simulink model "MSE452_Lab2_CHB_samplemodel"  (R2023a)
settings: Solver=ode23t  StartTime=0.0  StopTime=0.1  MaxStep=1e-5  RelTol=1e-3  EnableMultiTasking=on
InitFcn:
  | ma=0.99
  | f1=60
  | T1=1/f1
  | fs_ps=720
  | Ts_ps=1/fs_ps
  | fs_ls=4320
  | Ts_ls=1/fs_ls
values from neighbouring files (symbols this model uses):
  E = ratedOutputVoltage/3    (= 766.666666667)    [main.m]
  L = X / (2 * pi * ratedOutputFrequency)    [main.m]
  R = real(Z)    [main.m]
libraries: spsDCVoltageSourceLib x9, spsUniversalBridgeLib x9, spsTriangleGeneratorLib x9, spsVoltageMeasurementLib x5, spsSeriesRLCBranchLib x3, simulink x1, sps_lib x1
settings Model: Creator=jw  LastModifiedBy=auamai
settings SolverCC: AlgebraicLoopSolver=TrustRegion
settings DataIOCC: LimitDataPoints=on  SaveFormat=Array  SignalLoggingSaveFormat=ModelDataLogs  ReturnWorkspaceOutputs=off
settings OptimizationCC: InitFltsAndDblsToZero=on  LifeSpan=inf
settings DebuggingCC: SaveWithParameterizedLinksMsg=none  UnderspecifiedInitializationDetection=Classic  MergeDetectMultiDrivingBlocksExec=none  SignalResolutionControl=TryResolveAllWithWarning  SolverPrmCheckMsg=warning  MultiTaskDSMMsg=warning  MultiTaskCondExecSysMsg=none  FcnCallInpInsideContextMsg=warning  UnconnectedInputMsg=warning  UnconnectedOutputMsg=warning  UnconnectedLineMsg=warning  SFUnexpectedBacktrackingDiag=warning  SFNoUnconditionalDefaultTransitionDiag=warning  SFExecutionAtInitializationDiag=none  ArithmeticOperatorsInVariantConditions=warning
settings HardwareCC: ProdBitPerPointer=32  ProdBitPerSizeT=32  ProdBitPerPtrDiffT=32  ProdLargestAtomicFloat=None  ProdIntDivRoundTo=Undefined  ProdEndianess=Unspecified  ProdWordSize=32  ProdHWDeviceType=32-bit Generic
settings ModelReferenceCC: EnableRefExpFcnMdlSchedulingChecks=on  PropagateSignalLabelsOutOfModel=off
settings SFSimCC: CustomCodeUndefinedFunction=UseInterfaceOnly
settings CodeAppCC: StateflowObjectComments=on
settings GRTTargetCC: TargetFcnLib=ansi_tfl_tmw.mat  TargetLangStandard=C89/C90 (ANSI)  CombineOutputUpdateFcns=off  GRTInterface=on
settings ConfigComp: CovMetricSettings=dw  CovSaveCumulativeToWorkspaceVar=on  CovSaveSingleToWorkspaceVar=on

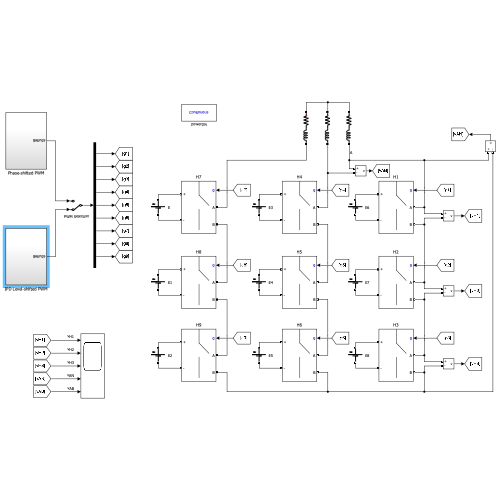
[thumbnail: Simulink's stored preview of the top-level diagram]
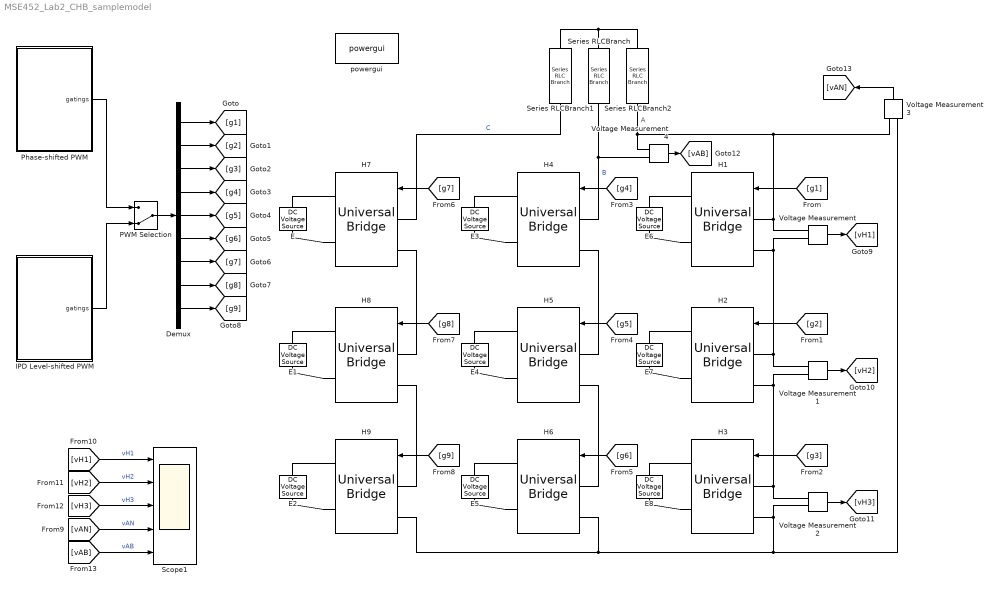
== system MSE452_Lab2_CHB_samplemodel ==
  note: A
  Demux : Demux  Outputs=9
  E{,1..8} (9 alike) : spsDCVoltageSourceLib/DC Voltage Source  Amplitude=E  Measurements=None
  H{1..9} (9 alike) : spsUniversalBridgeLib/Universal Bridge  Arms=2  SnubberResistance=1e5  SnubberCapacitance=inf  Device=Ideal Switches  Ron=1e-3  Lon=0  ForwardVoltages="[  0  0  ]"  ForwardVoltage=0  GTOparameters=[ 10e-6 , 20e-6 ]  IGBTparameters=[ 1e-6 , 2e-6 ]  Measurements=None  Measurements_2=None  converterType=Rectifier
  IPD Level-shifted PWM : Subsystem
  PWM Selection : ManualSwitch  CurrentSetting=0
  Phase-shifted PWM : Subsystem
  Scope1 : Scope  NumInputPorts=5
  Series RLCBranch : spsSeriesRLCBranchLib/Series RLC Branch  LConnTagsString=__new0  RConnTagsString=__new0  BranchType=RL  Resistance=R  Inductance=L  SetiL0=off  InitialCurrent=0  Capacitance=1e-6  Setx0=off  InitialVoltage=0  Measurements=None
  Series RLCBranch1 : spsSeriesRLCBranchLib/Series RLC Branch  LConnTagsString=__new0  RConnTagsString=__new0  BranchType=RL  Resistance=R  Inductance=L  SetiL0=off  InitialCurrent=0  Capacitance=1e-6  Setx0=off  InitialVoltage=0  Measurements=None
  Series RLCBranch2 : spsSeriesRLCBranchLib/Series RLC Branch  LConnTagsString=__new0  RConnTagsString=__new0  BranchType=RL  Resistance=R  Inductance=L  SetiL0=off  InitialCurrent=0  Capacitance=1e-6  Setx0=off  InitialVoltage=0  Measurements=None
  Voltage Measurement{,1..4} (5 alike) : spsVoltageMeasurementLib/Voltage Measurement  PhasorSimulation=off  OutputType=Complex  PSBequivalent=0
  powergui : sps_lib/powergui  Priority=1  SimulationMode=Continuous  SampleTime=50e-6  frequency=60  Iterations=50  frequencyindice=0  Pbase=100e6  ErrMax=1e-4  UnitsV=kV  UnitsW=MW  buscounter=0  FunctionMessages=off  echomessages=off  EnableUseOfTLC=off  CurrentSourceSwitches=off  DisableSnubberDevices=off  DisableRonSwitches=off  DisableVfSwitches=off  DisplayEquations=off  AutomaticDiscreteSolvers=off  SolverType=Tustin/Backward Euler (TBE)  Interpol=off  ExternalGateDelay=off  methode=off  Ts=100  x0status=blocks  SPID=on  SwTol=0  HookPort=off  NonlinearTolerance=1e-4  nMaxIteration=100  ContinueOnMaxIteration=off  RestoreLinks=warning  ResistiveCurrentMeasurement=off  Frange=[0:2:500]  Ylog=off  Xlog=on  ShowGrid=off  save=off  variable=ZData  structure=0  ZoomFFT=off  StartTime=0.0  cycles=1  DisplayStyle=1  fundamental=60  FreqAxis=off  MaxFrequency=1000  frequencyindicesteady=1  RmsSteady=1  display=off
  wires:
  [g1] -> H1/1
  [g2] -> H2/1
  [g3] -> H3/1
  [g4] -> H4/1
  [g5] -> H5/1
  [g6] -> H6/1
  [g7] -> H7/1
  [g8] -> H8/1
  [g9] -> H9/1
  Demux/1 -> [g1]
  Demux/2 -> [g2]
  Demux/3 -> [g3]
  Demux/4 -> [g4]
  Demux/5 -> [g5]
  Demux/6 -> [g6]
  Demux/7 -> [g7]
  Demux/8 -> [g8]
  Demux/9 -> [g9]
  Phase-shifted PWM/1(gatings) -> PWM Selection/1
  PWM Selection/1 -> Demux/1
  Voltage Measurement/1 -> [vH1]
  Voltage Measurement1/1 -> [vH2]
  Voltage Measurement2/1 -> [vH3]
  Voltage Measurement4/1 -> [vAB]
  Voltage Measurement3/1 -> [vAN]
  [vAN] -> Scope1/4  "vAN"
  [vH1] -> Scope1/1  "vH1"
  [vH2] -> Scope1/2  "vH2"
  [vH3] -> Scope1/3  "vH3"
  [vAB] -> Scope1/5  "vAB"
  IPD Level-shifted PWM/1(gatings) -> PWM Selection/2
  connections:
  H7/RConn2 -- E/LConn1
  E/RConn1 -- H7/RConn1
  E1/RConn1 -- H8/RConn1
  H8/RConn2 -- E1/LConn1
  E2/RConn1 -- H9/RConn1
  H9/RConn2 -- E2/LConn1
  H4/RConn2 -- E3/LConn1
  E5/RConn1 -- H6/RConn1
  E3/RConn1 -- H4/RConn1
  H6/RConn2 -- E5/LConn1
  E4/RConn1 -- H5/RConn1
  H5/RConn2 -- E4/LConn1
  H1/RConn2 -- E6/LConn1
  E8/RConn1 -- H3/RConn1
  E6/RConn1 -- H1/RConn1
  H3/RConn2 -- E8/LConn1
  E7/RConn1 -- H2/RConn1
  H2/RConn2 -- E7/LConn1
  H9/LConn2 -- H6/LConn2 -- H3/LConn2 -- Voltage Measurement2/LConn2 -- Voltage Measurement3/LConn2
  H9/LConn1 -- H8/LConn2
  H8/LConn1 -- H7/LConn2
  H4/LConn2 -- H5/LConn1
  H5/LConn2 -- H6/LConn1
  H1/LConn2 -- Voltage Measurement/LConn2 -- H2/LConn1 -- Voltage Measurement1/LConn1
  H2/LConn2 -- Voltage Measurement1/LConn2 -- H3/LConn1 -- Voltage Measurement2/LConn1
  H7/LConn1 -- Series RLCBranch1/RConn1  "C"
  Series RLCBranch/RConn1 -- H4/LConn1 -- Voltage Measurement4/LConn2  "B"
  H1/LConn1 -- Voltage Measurement/LConn1 -- Voltage Measurement3/LConn1 -- Series RLCBranch2/RConn1 -- Voltage Measurement4/LConn1
  Series RLCBranch1/LConn1 -- Series RLCBranch2/LConn1 -- Series RLCBranch/LConn1

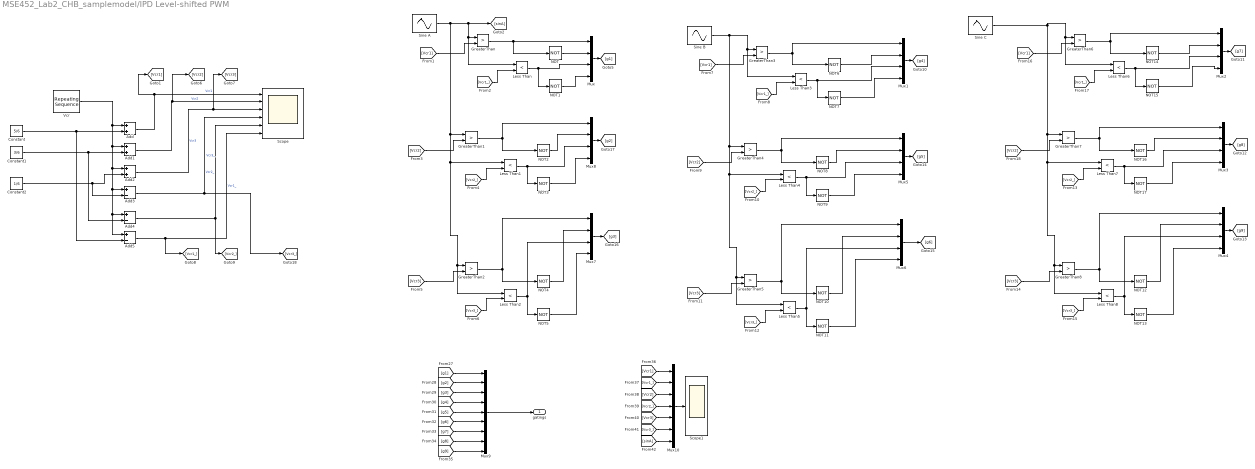
== system MSE452_Lab2_CHB_samplemodel/IPD Level-shifted PWM ==
  Add : Sum
  Add1 : Sum
  Add2 : Sum
  Add3 : Sum  Inputs=+-
  Add4 : Sum  Inputs=+-
  Add5 : Sum  Inputs=+-
  Constant : Constant  Value=5/6
  Constant1 : Constant  Value=3/6
  Constant2 : Constant  Value=1/6
  GreaterThan{,1..8} (9 alike) : RelationalOperator  Operator=>  OutDataTypeStr=boolean  RndMeth=Simplest  InputSameDT=off
  Less Than{,1..8} (9 alike) : RelationalOperator  Operator=<  OutDataTypeStr=boolean  RndMeth=Simplest  InputSameDT=off
  Mux{,1..8} (9 alike) : Mux
  Mux10 : Mux  Inputs=7
  Mux9 : Mux  Inputs=9
  NOT{,1..17} (18 alike) : Logic  Operator=NOT  IconShape=distinctive  AllPortsSameDT=off  OutDataTypeStr=boolean
  Scope : Scope  NumInputPorts=6
  Scope1 : Scope
  Sine A : Sin  Amplitude=0.25  Frequency=2*pi*f1  SampleTime=0
  Sine B : Sin  Amplitude=0.25  Frequency=2*pi*f1  Phase=-2/3*pi  SampleTime=0
  Sine C : Sin  Amplitude=0.25  Frequency=2*pi*f1  Phase=2/3*pi  SampleTime=0
  Vcr : simulink/Sources/Repeating Sequence  rep_seq_t=[0 1/4*Ts_ls 3/4*Ts_ls Ts_ls]  rep_seq_y=[0 1/6 -1/6 0]
  gatings : Outport  VectorParamsAs1DForOutWhenUnconnected=off
  wires:
  Mux9/1 -> gatings/1
  Mux/1 -> [g1]
  Mux1/1 -> [g4]
  Mux2/1 -> [g7]
  Mux3/1 -> [g8]
  Mux4/1 -> [g9]
  Mux5/1 -> [g5]
  Mux6/1 -> [g6]
  Mux7/1 -> [g3]
  Mux8/1 -> [g2]
  [g1] -> Mux9/1
  [g2] -> Mux9/2
  [g3] -> Mux9/3
  [g4] -> Mux9/4
  [g5] -> Mux9/5
  [g6] -> Mux9/6
  [g7] -> Mux9/7
  [g8] -> Mux9/8
  [g9] -> Mux9/9
  [Vcr1] -> Mux10/1
  [Vcr1_] -> Mux10/2
  [Vcr2] -> Mux10/3
  [Vcr2_] -> Mux10/4
  [Vcr3] -> Mux10/5
  [Vcr3_] -> Mux10/6
  Mux10/1 -> Scope1/1
  [sinA] -> Mux10/7
  Vcr/1 -> Add5/1, Add4/1, Add3/1, Add2/1, Add1/1, Add/1
  Constant/1 -> Add5/2, Add/2
  Add/1 -> [Vcr1], Scope/1  "Vcr1"
  Constant1/1 -> Add4/2, Add1/2
  Add1/1 -> [Vcr2], Scope/2  "Vcr2"
  Constant2/1 -> Add3/2, Add2/2
  Add2/1 -> [Vcr3], Scope/3  "Vcr3"
  Add5/1 -> [Vcr1_], Scope/6  "Vcr1_"
  Add3/1 -> [Vcr3_], Scope/4  "Vcr3_"
  Add4/1 -> [Vcr2_], Scope/5  "Vcr2_"
  [Vcr1] -> GreaterThan/2
  GreaterThan/1 -> NOT/1, Mux/1
  NOT/1 -> Mux/2
  [Vcr1_] -> Less Than/2
  Less Than/1 -> NOT1/1, Mux/3
  NOT1/1 -> Mux/4
  NOT2/1 -> Mux8/2
  [Vcr2_] -> Less Than1/2
  NOT3/1 -> Mux8/4
  Less Than1/1 -> Mux8/3, NOT3/1
  GreaterThan1/1 -> Mux8/1, NOT2/1
  [Vcr2] -> GreaterThan1/2
  GreaterThan2/1 -> Mux7/1, NOT4/1
  Less Than2/1 -> Mux7/3, NOT5/1
  [Vcr3_] -> Less Than2/2
  NOT5/1 -> Mux7/4
  [Vcr3] -> GreaterThan2/2
  Sine A/1 -> Less Than/1, GreaterThan/1, [sinA], Less Than1/1, Less Than2/1, GreaterThan2/1, GreaterThan1/1
  NOT4/1 -> Mux7/2
  NOT6/1 -> Mux1/2
  NOT11/1 -> Mux6/4
  Less Than5/1 -> Mux6/3, NOT11/1
  GreaterThan3/1 -> Mux1/1, NOT6/1
  Less Than4/1 -> Mux5/3, NOT9/1
  GreaterThan5/1 -> Mux6/1, NOT10/1
  [Vcr3] -> GreaterThan5/2
  [Vcr1_] -> Less Than3/2
  [Vcr2_] -> Less Than4/2
  [Vcr3_] -> Less Than5/2
  NOT10/1 -> Mux6/2
  [Vcr2] -> GreaterThan4/2
  Sine B/1 -> Less Than3/1, GreaterThan3/1, Less Than4/1, Less Than5/1, GreaterThan5/1, GreaterThan4/1
  GreaterThan4/1 -> Mux5/1, NOT8/1
  Less Than3/1 -> Mux1/3, NOT7/1
  NOT8/1 -> Mux5/2
  NOT9/1 -> Mux5/4
  NOT7/1 -> Mux1/4
  [Vcr1] -> GreaterThan3/2
  Less Than7/1 -> Mux3/3, NOT17/1
  GreaterThan6/1 -> Mux2/1, NOT14/1
  Less Than8/1 -> Mux4/3, NOT13/1
  [Vcr3_] -> Less Than8/2
  NOT13/1 -> Mux4/4
  [Vcr1] -> GreaterThan6/2
  Less Than6/1 -> Mux2/3, NOT15/1
  GreaterThan7/1 -> Mux3/1, NOT16/1
  NOT17/1 -> Mux3/4
  GreaterThan8/1 -> Mux4/1, NOT12/1
  [Vcr2] -> GreaterThan7/2
  [Vcr2_] -> Less Than7/2
  [Vcr3] -> GreaterThan8/2
  [Vcr1_] -> Less Than6/2
  Sine C/1 -> Less Than6/1, GreaterThan6/1, Less Than7/1, Less Than8/1, GreaterThan8/1, GreaterThan7/1
  NOT15/1 -> Mux2/4
  NOT12/1 -> Mux4/2
  NOT14/1 -> Mux2/2
  NOT16/1 -> Mux3/2

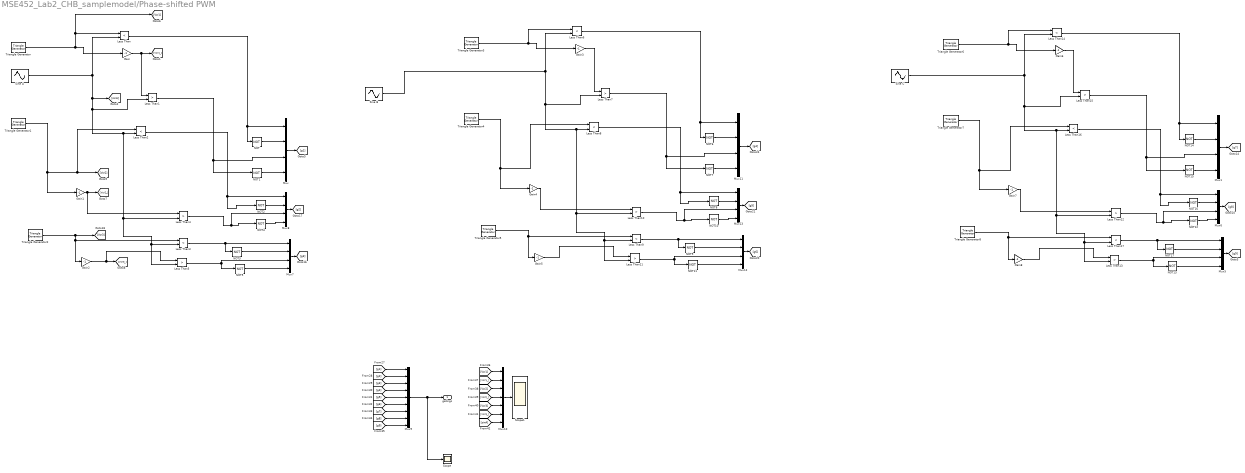
== system MSE452_Lab2_CHB_samplemodel/Phase-shifted PWM ==
  Gain{,1..8} (9 alike) : Gain  Gain=-1
  Less Than{,2..3,6,8..9,14,16..17} (9 alike) : RelationalOperator  Operator=<  OutDataTypeStr=boolean  RndMeth=Simplest  InputSameDT=off
  Less Than{1,4..5,7,10..13,15} (9 alike) : RelationalOperator  Operator=>  OutDataTypeStr=boolean  RndMeth=Simplest  InputSameDT=off
  Mux{,1,5..8,11..13} (9 alike) : Mux
  Mux10 : Mux  Inputs=7
  Mux9 : Mux  Inputs=9
  NOT{,1..17} (18 alike) : Logic  Operator=NOT  IconShape=distinctive  AllPortsSameDT=off  OutDataTypeStr=boolean
  Scope : Scope
  Scope1 : Scope
  Sine A : Sin  Amplitude=0.99  Frequency=2*pi*f1  SampleTime=0
  Sine B : Sin  Amplitude=0.99  Frequency=2*pi*f1  Phase=-2/3*pi  SampleTime=0
  Sine C : Sin  Amplitude=0.99  Frequency=2*pi*f1  Phase=2/3*pi  SampleTime=0
  Triangle Generator : spsTriangleGeneratorLib/Triangle Generator  Freq=fcr  Phase=90  Ts=0
  Triangle Generator1 : spsTriangleGeneratorLib/Triangle Generator  Freq=fcr  Phase=150  Ts=0
  Triangle Generator2 : spsTriangleGeneratorLib/Triangle Generator  Freq=fcr  Phase=210  Ts=0
  Triangle Generator3 : spsTriangleGeneratorLib/Triangle Generator  Freq=fcr  Phase=90  Ts=0
  Triangle Generator4 : spsTriangleGeneratorLib/Triangle Generator  Freq=fcr  Phase=150  Ts=0
  Triangle Generator5 : spsTriangleGeneratorLib/Triangle Generator  Freq=fcr  Phase=210  Ts=0
  Triangle Generator6 : spsTriangleGeneratorLib/Triangle Generator  Freq=fcr  Phase=90  Ts=0
  Triangle Generator7 : spsTriangleGeneratorLib/Triangle Generator  Freq=fcr  Phase=150  Ts=0
  Triangle Generator8 : spsTriangleGeneratorLib/Triangle Generator  Freq=fcr  Phase=210  Ts=0
  gatings : Outport  VectorParamsAs1DForOutWhenUnconnected=off
  wires:
  Mux9/1 -> Scope/1, gatings/1
  Sine A/1 -> Less Than4/2, Less Than5/2, Less Than3/2, Less Than2/2, Less Than1/2, [sinA], Less Than/2
  Mux/1 -> [g1]
  Mux7/1 -> [g3]
  Mux8/1 -> [g2]
  [g1] -> Mux9/1
  [g2] -> Mux9/2
  [g3] -> Mux9/3
  [g4] -> Mux9/4
  [g5] -> Mux9/5
  [g6] -> Mux9/6
  [g7] -> Mux9/7
  [g8] -> Mux9/8
  [g9] -> Mux9/9
  [Vcr1] -> Mux10/1
  [Vcr1_] -> Mux10/2
  [Vcr2] -> Mux10/3
  [Vcr2_] -> Mux10/4
  [Vcr3] -> Mux10/5
  [Vcr3_] -> Mux10/6
  Mux10/1 -> Scope1/1
  [sinA] -> Mux10/7
  Triangle Generator/1 -> Gain/1, Less Than/1, [Vcr1]
  Triangle Generator1/1 -> Less Than2/1, [Vcr2], Gain1/1
  Triangle Generator2/1 -> Gain2/1, Less Than3/1, [Vcr3]
  Gain/1 -> Less Than1/1, [Vcr1_]
  Gain1/1 -> Less Than4/1, [Vcr2_]
  Gain2/1 -> Less Than5/1, [Vcr3_]
  Less Than/1 -> NOT/1, Mux/1
  NOT/1 -> Mux/2
  Less Than1/1 -> NOT1/1, Mux/3
  NOT1/1 -> Mux/4
  Less Than2/1 -> NOT2/1, Mux8/1
  Less Than3/1 -> NOT3/1, Mux7/1
  NOT2/1 -> Mux8/2
  NOT3/1 -> Mux7/2
  Less Than4/1 -> NOT4/1, Mux8/3
  NOT4/1 -> Mux8/4
  Less Than5/1 -> NOT5/1, Mux7/3
  NOT5/1 -> Mux7/4
  Mux11/1 -> [g4]
  NOT9/1 -> Mux12/2
  Gain3/1 -> Less Than7/1
  NOT6/1 -> Mux11/2
  Mux12/1 -> [g6]
  NOT7/1 -> Mux11/4
  Triangle Generator4/1 -> Less Than8/1, Gain4/1
  Gain4/1 -> Less Than10/1
  Triangle Generator5/1 -> Gain5/1, Less Than9/1
  Less Than6/1 -> NOT6/1, Mux11/1
  Mux13/1 -> [g5]
  Less Than7/1 -> NOT7/1, Mux11/3
  Gain5/1 -> Less Than11/1
  Sine B/1 -> Less Than10/2, Less Than11/2, Less Than9/2, Less Than8/2, Less Than7/2, Less Than6/2
  NOT11/1 -> Mux12/4
  Triangle Generator3/1 -> Gain3/1, Less Than6/1
  Less Than11/1 -> NOT11/1, Mux12/3
  NOT10/1 -> Mux13/4
  Less Than9/1 -> NOT9/1, Mux12/1
  Less Than10/1 -> NOT10/1, Mux13/3
  Less Than8/1 -> NOT8/1, Mux13/1
  NOT8/1 -> Mux13/2
  Sine C/1 -> Less Than14/2, Less Than12/2, Less Than13/2, Less Than17/2, Less Than16/2, Less Than15/2
  Triangle Generator7/1 -> Less Than16/1, Gain7/1
  Gain8/1 -> Less Than13/1
  Less Than16/1 -> NOT16/1, Mux6/1
  NOT12/1 -> Mux6/4
  Gain6/1 -> Less Than15/1
  Triangle Generator6/1 -> Gain6/1, Less Than14/1
  NOT14/1 -> Mux1/2
  Less Than13/1 -> NOT13/1, Mux5/3
  Less Than12/1 -> NOT12/1, Mux6/3
  NOT13/1 -> Mux5/4
  Gain7/1 -> Less Than12/1
  Less Than14/1 -> NOT14/1, Mux1/1
  Mux6/1 -> [g8]
  NOT16/1 -> Mux6/2
  Triangle Generator8/1 -> Gain8/1, Less Than17/1
  NOT15/1 -> Mux1/4
  Less Than17/1 -> NOT17/1, Mux5/1
  Mux5/1 -> [g9]
  Less Than15/1 -> NOT15/1, Mux1/3
  NOT17/1 -> Mux5/2
  Mux1/1 -> [g7]
